simulink model "SystemDrivers"  (Simulink 8.3)
settings: Solver=ode45  StartTime=0.0  StopTime=50  RelTol=1e-4
model workspace (MAT data in the model file):
  MPS_ModuleName = 'ACC_Enhancement.ECR'
  variantInfo = VariabilitySupport
  variantInfo.name = 'ACCVarModel'
  variantInfo.featureModels = FeatureModel
  variantInfo.featureModels.id = '7NIE1o_FUkv'
  variantInfo.featureModels.name = 'ACCVars'
  variantInfo.featureModels.root = Feature
  variantInfo.featureModels.root.id = '7NIE1o_FUkw'
  variantInfo.featureModels.root.children(1) = Feature
  variantInfo.featureModels.root.children(1).id = '7NIE1o_FUxh'
  variantInfo.featureModels.root.children(1).name = 'SubjectProdFunction'
  variantInfo.featureModels.root.children(1).children(1) = Feature
  variantInfo.featureModels.root.children(1).children(1).id = '7NIE1o_FUzk'
  variantInfo.featureModels.root.children(1).children(1).name = 'S_ACC'
  variantInfo.featureModels.root.children(1).children(2) = Feature
  variantInfo.featureModels.root.children(1).children(2).id = '23v$6Q_kdyy'
  variantInfo.featureModels.root.children(1).children(2).name = 'S_ACC_SF'
  variantInfo.featureModels.root.children(1).children(3) = Feature
  variantInfo.featureModels.root.children(1).children(3).id = '7NIE1o_FUzr'
  variantInfo.featureModels.root.children(1).children(3).name = 'S_LearningACC'
  variantInfo.featureModels.root.children(1).children(4) = Feature
  variantInfo.featureModels.root.children(1).children(4).id = '23v$6Q_kdyD'
  variantInfo.featureModels.root.children(1).children(4).name = 'S_LearningACC_SF'
  variantInfo.featureModels.root.children(2) = Feature
  variantInfo.featureModels.root.children(2).id = '64YhESPcT$J'
  variantInfo.featureModels.root.children(2).name = 'SubjectDriverType'
  variantInfo.featureModels.root.children(2).children(1) = Feature
  variantInfo.featureModels.root.children(2).children(1).id = '64YhESPcT$S'
  variantInfo.featureModels.root.children(2).children(1).name = 'S_NormalDriver'
  variantInfo.featureModels.root.children(2).children(2) = Feature
  variantInfo.featureModels.root.children(2).children(2).id = '64YhESPcT$V'
  variantInfo.featureModels.root.children(2).children(2).name = 'S_ErraticDriver'
  variantInfo.featureModels.root.children(3) = Feature
  variantInfo.featureModels.root.children(3).id = '64YhESPd24W'
  variantInfo.featureModels.root.children(3).name = 'TargetProdFunction'
  variantInfo.featureModels.root.children(3).children(1) = Feature
  variantInfo.featureModels.root.children(3).children(1).id = '64YhESPd24Y'
  variantInfo.featureModels.root.children(3).children(1).name = 'T_ACC'
  variantInfo.featureModels.root.children(3).children(2) = Feature
  variantInfo.featureModels.root.children(3).children(2).id = '64YhESPd24Z'
  variantInfo.featureModels.root.children(3).children(2).name = 'T_LearningACC'
  variantInfo.featureModels.root.children(4) = Feature
  variantInfo.featureModels.root.children(4).id = '64YhESPd250'
  variantInfo.featureModels.root.children(4).name = 'TargetDriverType'
  variantInfo.featureModels.root.children(4).children(1) = Feature
  variantInfo.featureModels.root.children(4).children(1).id = '64YhESPd252'
  variantInfo.featureModels.root.children(4).children(1).name = 'T_NormalDriver'
  variantInfo.featureModels.root.children(4).children(2) = Feature
  variantInfo.featureModels.root.children(4).children(2).id = '64YhESPd253'
  variantInfo.featureModels.root.children(4).children(2).name = 'T_ErraticDriver'
  variantInfo.configModels(1) = VariantConfigurationModel
  variantInfo.configModels(1).id = '7NIE1o_G2gu'
  variantInfo.configModels(1).name = 'NormalACC'
  variantInfo.configModels(1).featureRef = MpsObjectRef
  variantInfo.configModels(1).featureRef.targetNodeId = '7NIE1o_FUkv'
  variantInfo.configModels(1).featureRef.resolveInfo = 'ACCVars'
  variantInfo.configModels(1).rootFeature = VariantSelectedFeature
  variantInfo.configModels(1).rootFeature.featureRef = MpsObjectRef
  variantInfo.configModels(1).rootFeature.featureRef.targetNodeId = '7NIE1o_FUkw'
  variantInfo.configModels(1).rootFeature.featureRef.resolveInfo = 'ACCVars_root'
  variantInfo.configModels(1).rootFeature.children(1) = VariantSelectedFeature
  variantInfo.configModels(1).rootFeature.children(1).featureRef = MpsObjectRef
  variantInfo.configModels(1).rootFeature.children(1).featureRef.targetNodeId = '7NIE1o_FUxh'
  variantInfo.configModels(1).rootFeature.children(1).featureRef.resolveInfo = 'SubjectProdFunction'
  variantInfo.configModels(1).rootFeature.children(1).children = VariantSelectedFeature
  variantInfo.configModels(1).rootFeature.children(1).children.featureRef = MpsObjectRef
  variantInfo.configModels(1).rootFeature.children(1).children.featureRef.targetNodeId = '7NIE1o_FUzk'
  variantInfo.configModels(1).rootFeature.children(1).children.featureRef.resolveInfo = 'S_ACC'
  variantInfo.configModels(1).rootFeature.children(2) = VariantSelectedFeature
  variantInfo.configModels(1).rootFeature.children(2).featureRef = MpsObjectRef
  variantInfo.configModels(1).rootFeature.children(2).featureRef.targetNodeId = '64YhESPcT$J'
  variantInfo.configModels(1).rootFeature.children(2).featureRef.resolveInfo = 'SubjectDriverType'
  variantInfo.configModels(1).rootFeature.children(2).children = VariantSelectedFeature
  variantInfo.configModels(1).rootFeature.children(2).children.featureRef = MpsObjectRef
  variantInfo.configModels(1).rootFeature.children(2).children.featureRef.targetNodeId = '64YhESPcT$S'
  variantInfo.configModels(1).rootFeature.children(2).children.featureRef.resolveInfo = 'S_NormalDriver'
  variantInfo.configModels(1).rootFeature.children(3) = VariantSelectedFeature
  variantInfo.configModels(1).rootFeature.children(3).featureRef = MpsObjectRef
  variantInfo.configModels(1).rootFeature.children(3).featureRef.targetNodeId = '64YhESPd24W'
  variantInfo.configModels(1).rootFeature.children(3).featureRef.resolveInfo = 'TargetProdFunction'
  variantInfo.configModels(1).rootFeature.children(3).children = VariantSelectedFeature
  variantInfo.configModels(1).rootFeature.children(3).children.featureRef = MpsObjectRef
  variantInfo.configModels(1).rootFeature.children(3).children.featureRef.targetNodeId = '64YhESPd24Y'
  variantInfo.configModels(1).rootFeature.children(3).children.featureRef.resolveInfo = 'T_ACC'
  variantInfo.configModels(1).rootFeature.children(4) = VariantSelectedFeature
  variantInfo.configModels(1).rootFeature.children(4).featureRef = MpsObjectRef
  variantInfo.configModels(1).rootFeature.children(4).featureRef.targetNodeId = '64YhESPd250'
  variantInfo.configModels(1).rootFeature.children(4).featureRef.resolveInfo = 'TargetDriverType'
  variantInfo.configModels(1).rootFeature.children(4).children = VariantSelectedFeature
  variantInfo.configModels(1).rootFeature.children(4).children.featureRef = MpsObjectRef
  variantInfo.configModels(1).rootFeature.children(4).children.featureRef.targetNodeId = '64YhESPd252'
  variantInfo.configModels(1).rootFeature.children(4).children.featureRef.resolveInfo = 'T_NormalDriver'
  variantInfo.configModels(2) = VariantConfigurationModel
  variantInfo.configModels(2).id = '23v$6Q_kdSe'
  variantInfo.configModels(2).name = 'NormalACC_SF'
  variantInfo.configModels(2).featureRef = MpsObjectRef
  variantInfo.configModels(2).featureRef.targetNodeId = '7NIE1o_FUkv'
  variantInfo.configModels(2).featureRef.resolveInfo = 'ACCVars'
  variantInfo.configModels(2).rootFeature = VariantSelectedFeature
  variantInfo.configModels(2).rootFeature.featureRef = MpsObjectRef
  variantInfo.configModels(2).rootFeature.featureRef.targetNodeId = '7NIE1o_FUkw'
  variantInfo.configModels(2).rootFeature.featureRef.resolveInfo = 'ACCVars_root'
  variantInfo.configModels(2).rootFeature.children(1) = VariantSelectedFeature
  variantInfo.configModels(2).rootFeature.children(1).featureRef = MpsObjectRef
  variantInfo.configModels(2).rootFeature.children(1).featureRef.targetNodeId = '7NIE1o_FUxh'
  variantInfo.configModels(2).rootFeature.children(1).featureRef.resolveInfo = 'SubjectProdFunction'
  variantInfo.configModels(2).rootFeature.children(1).children = VariantSelectedFeature
  variantInfo.configModels(2).rootFeature.children(1).children.featureRef = MpsObjectRef
  variantInfo.configModels(2).rootFeature.children(1).children.featureRef.targetNodeId = '23v$6Q_kdyy'
  variantInfo.configModels(2).rootFeature.children(1).children.featureRef.resolveInfo = 'S_ACC_SF'
  variantInfo.configModels(2).rootFeature.children(2) = VariantSelectedFeature
  variantInfo.configModels(2).rootFeature.children(2).featureRef = MpsObjectRef
  variantInfo.configModels(2).rootFeature.children(2).featureRef.targetNodeId = '64YhESPcT$J'
  variantInfo.configModels(2).rootFeature.children(2).featureRef.resolveInfo = 'SubjectDriverType'
  variantInfo.configModels(2).rootFeature.children(2).children = VariantSelectedFeature
  variantInfo.configModels(2).rootFeature.children(2).children.featureRef = MpsObjectRef
  variantInfo.configModels(2).rootFeature.children(2).children.featureRef.targetNodeId = '64YhESPcT$S'
  variantInfo.configModels(2).rootFeature.children(2).children.featureRef.resolveInfo = 'S_NormalDriver'
  variantInfo.configModels(2).rootFeature.children(3) = VariantSelectedFeature
  variantInfo.configModels(2).rootFeature.children(3).featureRef = MpsObjectRef
  variantInfo.configModels(2).rootFeature.children(3).featureRef.targetNodeId = '64YhESPd24W'
  variantInfo.configModels(2).rootFeature.children(3).featureRef.resolveInfo = 'TargetProdFunction'
  variantInfo.configModels(2).rootFeature.children(3).children = VariantSelectedFeature
  variantInfo.configModels(2).rootFeature.children(3).children.featureRef = MpsObjectRef
  variantInfo.configModels(2).rootFeature.children(3).children.featureRef.targetNodeId = '64YhESPd24Y'
  variantInfo.configModels(2).rootFeature.children(3).children.featureRef.resolveInfo = 'T_ACC'
  variantInfo.configModels(2).rootFeature.children(4) = VariantSelectedFeature
  variantInfo.configModels(2).rootFeature.children(4).featureRef = MpsObjectRef
  variantInfo.configModels(2).rootFeature.children(4).featureRef.targetNodeId = '64YhESPd250'
  variantInfo.configModels(2).rootFeature.children(4).featureRef.resolveInfo = 'TargetDriverType'
  variantInfo.configModels(2).rootFeature.children(4).children = VariantSelectedFeature
  variantInfo.configModels(2).rootFeature.children(4).children.featureRef = MpsObjectRef
  variantInfo.configModels(2).rootFeature.children(4).children.featureRef.targetNodeId = '64YhESPd252'
  variantInfo.configModels(2).rootFeature.children(4).children.featureRef.resolveInfo = 'T_NormalDriver'
  variantInfo.configModels(3) = VariantConfigurationModel
  variantInfo.configModels(3).id = '7NIE1o_FUDp'
  variantInfo.configModels(3).name = 'ErraticDriverACC'
  variantInfo.configModels(3).featureRef = MpsObjectRef
  variantInfo.configModels(3).featureRef.targetNodeId = '7NIE1o_FUkv'
  variantInfo.configModels(3).featureRef.resolveInfo = 'ACCVars'
  variantInfo.configModels(3).rootFeature = VariantSelectedFeature
  variantInfo.configModels(3).rootFeature.featureRef = MpsObjectRef
  variantInfo.configModels(3).rootFeature.featureRef.targetNodeId = '7NIE1o_FUkw'
  variantInfo.configModels(3).rootFeature.featureRef.resolveInfo = 'ACCVars_root'
  variantInfo.configModels(3).rootFeature.children(1) = VariantSelectedFeature
  variantInfo.configModels(3).rootFeature.children(1).featureRef = MpsObjectRef
  variantInfo.configModels(3).rootFeature.children(1).featureRef.targetNodeId = '7NIE1o_FUxh'
  variantInfo.configModels(3).rootFeature.children(1).featureRef.resolveInfo = 'SubjectProdFunction'
  variantInfo.configModels(3).rootFeature.children(1).children = VariantSelectedFeature
  variantInfo.configModels(3).rootFeature.children(1).children.featureRef = MpsObjectRef
  variantInfo.configModels(3).rootFeature.children(1).children.featureRef.targetNodeId = '7NIE1o_FUzk'
  variantInfo.configModels(3).rootFeature.children(1).children.featureRef.resolveInfo = 'S_ACC'
  variantInfo.configModels(3).rootFeature.children(2) = VariantSelectedFeature
  variantInfo.configModels(3).rootFeature.children(2).featureRef = MpsObjectRef
  variantInfo.configModels(3).rootFeature.children(2).featureRef.targetNodeId = '64YhESPcT$J'
  variantInfo.configModels(3).rootFeature.children(2).featureRef.resolveInfo = 'SubjectDriverType'
  variantInfo.configModels(3).rootFeature.children(2).children = VariantSelectedFeature
  variantInfo.configModels(3).rootFeature.children(2).children.featureRef = MpsObjectRef
  variantInfo.configModels(3).rootFeature.children(2).children.featureRef.targetNodeId = '64YhESPcT$S'
  variantInfo.configModels(3).rootFeature.children(2).children.featureRef.resolveInfo = 'S_NormalDriver'
  variantInfo.configModels(3).rootFeature.children(3) = VariantSelectedFeature
  variantInfo.configModels(3).rootFeature.children(3).featureRef = MpsObjectRef
  variantInfo.configModels(3).rootFeature.children(3).featureRef.targetNodeId = '64YhESPd24W'
  variantInfo.configModels(3).rootFeature.children(3).featureRef.resolveInfo = 'TargetProdFunction'
  variantInfo.configModels(3).rootFeature.children(3).children = VariantSelectedFeature
  variantInfo.configModels(3).rootFeature.children(3).children.featureRef = MpsObjectRef
  variantInfo.configModels(3).rootFeature.children(3).children.featureRef.targetNodeId = '64YhESPd24Y'
  variantInfo.configModels(3).rootFeature.children(3).children.featureRef.resolveInfo = 'T_ACC'
  variantInfo.configModels(3).rootFeature.children(4) = VariantSelectedFeature
  variantInfo.configModels(3).rootFeature.children(4).featureRef = MpsObjectRef
  variantInfo.configModels(3).rootFeature.children(4).featureRef.targetNodeId = '64YhESPd250'
  variantInfo.configModels(3).rootFeature.children(4).featureRef.resolveInfo = 'TargetDriverType'
  variantInfo.configModels(3).rootFeature.children(4).children = VariantSelectedFeature
  variantInfo.configModels(3).rootFeature.children(4).children.featureRef = MpsObjectRef
  variantInfo.configModels(3).rootFeature.children(4).children.featureRef.targetNodeId = '64YhESPd253'
  variantInfo.configModels(3).rootFeature.children(4).children.featureRef.resolveInfo = 'T_ErraticDriver'
  variantInfo.configModels(4) = VariantConfigurationModel
  variantInfo.configModels(4).id = '23v$6Q_kef3'
  variantInfo.configModels(4).name = 'ErraticDriverACC_SF'
  variantInfo.configModels(4).featureRef = MpsObjectRef
  variantInfo.configModels(4).featureRef.targetNodeId = '7NIE1o_FUkv'
  variantInfo.configModels(4).featureRef.resolveInfo = 'ACCVars'
  variantInfo.configModels(4).rootFeature = VariantSelectedFeature
  variantInfo.configModels(4).rootFeature.featureRef = MpsObjectRef
  variantInfo.configModels(4).rootFeature.featureRef.targetNodeId = '7NIE1o_FUkw'
  variantInfo.configModels(4).rootFeature.featureRef.resolveInfo = 'ACCVars_root'
  variantInfo.configModels(4).rootFeature.children(1) = VariantSelectedFeature
  variantInfo.configModels(4).rootFeature.children(1).featureRef = MpsObjectRef
  variantInfo.configModels(4).rootFeature.children(1).featureRef.targetNodeId = '7NIE1o_FUxh'
  variantInfo.configModels(4).rootFeature.children(1).featureRef.resolveInfo = 'SubjectProdFunction'
  variantInfo.configModels(4).rootFeature.children(1).children = VariantSelectedFeature
  variantInfo.configModels(4).rootFeature.children(1).children.featureRef = MpsObjectRef
  variantInfo.configModels(4).rootFeature.children(1).children.featureRef.targetNodeId = '23v$6Q_kdyy'
  variantInfo.configModels(4).rootFeature.children(1).children.featureRef.resolveInfo = 'S_ACC_SF'
  variantInfo.configModels(4).rootFeature.children(2) = VariantSelectedFeature
  variantInfo.configModels(4).rootFeature.children(2).featureRef = MpsObjectRef
  variantInfo.configModels(4).rootFeature.children(2).featureRef.targetNodeId = '64YhESPcT$J'
  variantInfo.configModels(4).rootFeature.children(2).featureRef.resolveInfo = 'SubjectDriverType'
  variantInfo.configModels(4).rootFeature.children(2).children = VariantSelectedFeature
  variantInfo.configModels(4).rootFeature.children(2).children.featureRef = MpsObjectRef
  variantInfo.configModels(4).rootFeature.children(2).children.featureRef.targetNodeId = '64YhESPcT$S'
  variantInfo.configModels(4).rootFeature.children(2).children.featureRef.resolveInfo = 'S_NormalDriver'
  variantInfo.configModels(4).rootFeature.children(3) = VariantSelectedFeature
  variantInfo.configModels(4).rootFeature.children(3).featureRef = MpsObjectRef
  variantInfo.configModels(4).rootFeature.children(3).featureRef.targetNodeId = '64YhESPd24W'
  variantInfo.configModels(4).rootFeature.children(3).featureRef.resolveInfo = 'TargetProdFunction'
  variantInfo.configModels(4).rootFeature.children(3).children = VariantSelectedFeature
  variantInfo.configModels(4).rootFeature.children(3).children.featureRef = MpsObjectRef
  variantInfo.configModels(4).rootFeature.children(3).children.featureRef.targetNodeId = '64YhESPd24Y'
  variantInfo.configModels(4).rootFeature.children(3).children.featureRef.resolveInfo = 'T_ACC'
  variantInfo.configModels(4).rootFeature.children(4) = VariantSelectedFeature
  variantInfo.configModels(4).rootFeature.children(4).featureRef = MpsObjectRef
  variantInfo.configModels(4).rootFeature.children(4).featureRef.targetNodeId = '64YhESPd250'
  variantInfo.configModels(4).rootFeature.children(4).featureRef.resolveInfo = 'TargetDriverType'
  variantInfo.configModels(4).rootFeature.children(4).children = VariantSelectedFeature
  variantInfo.configModels(4).rootFeature.children(4).children.featureRef = MpsObjectRef
  variantInfo.configModels(4).rootFeature.children(4).children.featureRef.targetNodeId = '64YhESPd253'
  variantInfo.configModels(4).rootFeature.children(4).children.featureRef.resolveInfo = 'T_ErraticDriver'
  variantInfo.configModels(5) = VariantConfigurationModel
  variantInfo.configModels(5).id = '7NIE1o_FUF3'
  variantInfo.configModels(5).name = 'ErraticDriverACCFix'
  variantInfo.configModels(5).featureRef = MpsObjectRef
  variantInfo.configModels(5).featureRef.targetNodeId = '7NIE1o_FUkv'
  variantInfo.configModels(5).featureRef.resolveInfo = 'ACCVars'
  variantInfo.configModels(5).rootFeature = VariantSelectedFeature
  variantInfo.configModels(5).rootFeature.featureRef = MpsObjectRef
  variantInfo.configModels(5).rootFeature.featureRef.targetNodeId = '7NIE1o_FUkw'
  variantInfo.configModels(5).rootFeature.featureRef.resolveInfo = 'ACCVars_root'
  variantInfo.configModels(5).rootFeature.children(1) = VariantSelectedFeature
  variantInfo.configModels(5).rootFeature.children(1).featureRef = MpsObjectRef
  variantInfo.configModels(5).rootFeature.children(1).featureRef.targetNodeId = '7NIE1o_FUxh'
  variantInfo.configModels(5).rootFeature.children(1).featureRef.resolveInfo = 'SubjectProdFunction'
  variantInfo.configModels(5).rootFeature.children(1).children = VariantSelectedFeature
  variantInfo.configModels(5).rootFeature.children(1).children.featureRef = MpsObjectRef
  variantInfo.configModels(5).rootFeature.children(1).children.featureRef.targetNodeId = '7NIE1o_FUzr'
  variantInfo.configModels(5).rootFeature.children(1).children.featureRef.resolveInfo = 'S_LearningACC'
  variantInfo.configModels(5).rootFeature.children(2) = VariantSelectedFeature
  variantInfo.configModels(5).rootFeature.children(2).featureRef = MpsObjectRef
  variantInfo.configModels(5).rootFeature.children(2).featureRef.targetNodeId = '64YhESPcT$J'
  variantInfo.configModels(5).rootFeature.children(2).featureRef.resolveInfo = 'SubjectDriverType'
  variantInfo.configModels(5).rootFeature.children(2).children = VariantSelectedFeature
  variantInfo.configModels(5).rootFeature.children(2).children.featureRef = MpsObjectRef
  variantInfo.configModels(5).rootFeature.children(2).children.featureRef.targetNodeId = '64YhESPcT$S'
  variantInfo.configModels(5).rootFeature.children(2).children.featureRef.resolveInfo = 'S_NormalDriver'
  variantInfo.configModels(5).rootFeature.children(3) = VariantSelectedFeature
  variantInfo.configModels(5).rootFeature.children(3).featureRef = MpsObjectRef
  variantInfo.configModels(5).rootFeature.children(3).featureRef.targetNodeId = '64YhESPd24W'
  variantInfo.configModels(5).rootFeature.children(3).featureRef.resolveInfo = 'TargetProdFunction'
  variantInfo.configModels(5).rootFeature.children(3).children = VariantSelectedFeature
  variantInfo.configModels(5).rootFeature.children(3).children.featureRef = MpsObjectRef
  variantInfo.configModels(5).rootFeature.children(3).children.featureRef.targetNodeId = '64YhESPd24Y'
  variantInfo.configModels(5).rootFeature.children(3).children.featureRef.resolveInfo = 'T_ACC'
  variantInfo.configModels(5).rootFeature.children(4) = VariantSelectedFeature
  variantInfo.configModels(5).rootFeature.children(4).featureRef = MpsObjectRef
  variantInfo.configModels(5).rootFeature.children(4).featureRef.targetNodeId = '64YhESPd250'
  variantInfo.configModels(5).rootFeature.children(4).featureRef.resolveInfo = 'TargetDriverType'
  variantInfo.configModels(5).rootFeature.children(4).children = VariantSelectedFeature
  variantInfo.configModels(5).rootFeature.children(4).children.featureRef = MpsObjectRef
  variantInfo.configModels(5).rootFeature.children(4).children.featureRef.targetNodeId = '64YhESPd253'
  variantInfo.configModels(5).rootFeature.children(4).children.featureRef.resolveInfo = 'T_ErraticDriver'
  variantInfo.configModels(6) = VariantConfigurationModel
  variantInfo.configModels(6).id = '23v$6Q_kdWi'
  variantInfo.configModels(6).name = 'ErraticDriverACCFix_SF'
  variantInfo.configModels(6).featureRef = MpsObjectRef
  variantInfo.configModels(6).featureRef.targetNodeId = '7NIE1o_FUkv'
  variantInfo.configModels(6).featureRef.resolveInfo = 'ACCVars'
  variantInfo.configModels(6).rootFeature = VariantSelectedFeature
  variantInfo.configModels(6).rootFeature.featureRef = MpsObjectRef
  variantInfo.configModels(6).rootFeature.featureRef.targetNodeId = '7NIE1o_FUkw'
  variantInfo.configModels(6).rootFeature.featureRef.resolveInfo = 'ACCVars_root'
  variantInfo.configModels(6).rootFeature.children(1) = VariantSelectedFeature
  variantInfo.configModels(6).rootFeature.children(1).featureRef = MpsObjectRef
  variantInfo.configModels(6).rootFeature.children(1).featureRef.targetNodeId = '7NIE1o_FUxh'
  variantInfo.configModels(6).rootFeature.children(1).featureRef.resolveInfo = 'SubjectProdFunction'
  variantInfo.configModels(6).rootFeature.children(1).children = VariantSelectedFeature
  variantInfo.configModels(6).rootFeature.children(1).children.featureRef = MpsObjectRef
  variantInfo.configModels(6).rootFeature.children(1).children.featureRef.targetNodeId = '23v$6Q_kdyD'
  variantInfo.configModels(6).rootFeature.children(1).children.featureRef.resolveInfo = 'S_LearningACC_SF'
  variantInfo.configModels(6).rootFeature.children(2) = VariantSelectedFeature
  variantInfo.configModels(6).rootFeature.children(2).featureRef = MpsObjectRef
  variantInfo.configModels(6).rootFeature.children(2).featureRef.targetNodeId = '64YhESPcT$J'
  variantInfo.configModels(6).rootFeature.children(2).featureRef.resolveInfo = 'SubjectDriverType'
  variantInfo.configModels(6).rootFeature.children(2).children = VariantSelectedFeature
  variantInfo.configModels(6).rootFeature.children(2).children.featureRef = MpsObjectRef
  variantInfo.configModels(6).rootFeature.children(2).children.featureRef.targetNodeId = '64YhESPcT$S'
  variantInfo.configModels(6).rootFeature.children(2).children.featureRef.resolveInfo = 'S_NormalDriver'
  variantInfo.configModels(6).rootFeature.children(3) = VariantSelectedFeature
  variantInfo.configModels(6).rootFeature.children(3).featureRef = MpsObjectRef
  variantInfo.configModels(6).rootFeature.children(3).featureRef.targetNodeId = '64YhESPd24W'
  variantInfo.configModels(6).rootFeature.children(3).featureRef.resolveInfo = 'TargetProdFunction'
  variantInfo.configModels(6).rootFeature.children(3).children = VariantSelectedFeature
  variantInfo.configModels(6).rootFeature.children(3).children.featureRef = MpsObjectRef
  variantInfo.configModels(6).rootFeature.children(3).children.featureRef.targetNodeId = '64YhESPd24Y'
  variantInfo.configModels(6).rootFeature.children(3).children.featureRef.resolveInfo = 'T_ACC'
  variantInfo.configModels(6).rootFeature.children(4) = VariantSelectedFeature
  variantInfo.configModels(6).rootFeature.children(4).featureRef = MpsObjectRef
  variantInfo.configModels(6).rootFeature.children(4).featureRef.targetNodeId = '64YhESPd250'
  variantInfo.configModels(6).rootFeature.children(4).featureRef.resolveInfo = 'TargetDriverType'
  variantInfo.configModels(6).rootFeature.children(4).children = VariantSelectedFeature
  variantInfo.configModels(6).rootFeature.children(4).children.featureRef = MpsObjectRef
  variantInfo.configModels(6).rootFeature.children(4).children.featureRef.targetNodeId = '64YhESPd253'
  variantInfo.configModels(6).rootFeature.children(4).children.featureRef.resolveInfo = 'T_ErraticDriver'
undefined symbols (not defined in the file): Engine, Trans
libraries: simulink x2
settings Model: Creator=swami  LastModifiedBy=swami
settings SolverCC: ShapePreserveControl=EnableAll  ZeroCrossControl=EnableAll
settings DataIOCC: SignalLoggingSaveFormat=Dataset
settings DebuggingCC: UnderspecifiedInitializationDetection=Simplified  MergeDetectMultiDrivingBlocksExec=error  FrameProcessingCompatibilityMsg=error  StateNameClashWarn=none
settings ModelReferenceCC: UpdateModelReferenceTargets=Force
settings GRTTargetCC: CombineOutputUpdateFcns=on  GRTInterface=off
settings ConfigComp: CovMetricSettings=dw  CovHtmlReporting=on  CovSaveCumulativeToWorkspaceVar=on  CovSaveSingleToWorkspaceVar=on  CovModelRefEnable=Off  CovExternalEMLEnable=off  CovSFcnEnable=off

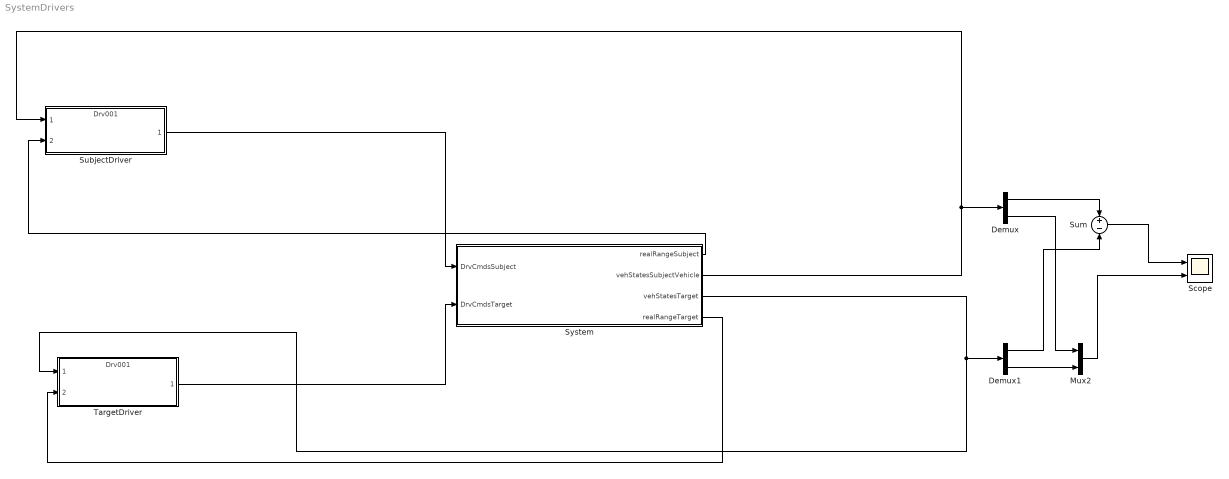
== system SystemDrivers ==
  Demux : Demux  Outputs=2
  Demux1 : Demux  Outputs=2
  Mux2 : Mux  Inputs=2
  Scope : Scope  NumInputPorts=2
  SubjectDriver : ModelReference  ModelNameDialog=Drv001  ParameterArgumentNames=pDrv  ParameterArgumentValues=DrvSubject  SimulationMode=Normal  Variant=on  OverrideUsingVariant=ECR1_varDrv001  ModelReferenceVersion=1.22  CopyOfModelName=Drv001  DefaultDataLogging=on
      settings: AttributesFormatString=%<ActiveVariant>
  Sum : Sum  Inputs=+-
  System : Subsystem
  TargetDriver : ModelReference  ModelNameDialog=Drv001  ParameterArgumentNames=pDrv  ParameterArgumentValues=DrvTarget  SimulationMode=Normal  Variant=on  OverrideUsingVariant=ECR1_varDrv001  ModelReferenceVersion=1.22  CopyOfModelName=Drv001  DefaultDataLogging=on
      settings: AttributesFormatString=%<ActiveVariant>
  wires:
  Demux/1 -> Sum/1
  Demux1/1 -> Sum/2
  Demux/2 -> Mux2/1
  Demux1/2 -> Mux2/2
  Mux2/1 -> Scope/2
  Sum/1 -> Scope/1
  System/2(vehStatesSubjectVehicle) -> SubjectDriver/1, Demux/1
  SubjectDriver/1 -> System/1(DrvCmdsSubject)
  TargetDriver/1 -> System/2(DrvCmdsTarget)
  System/1(realRangeSubject) -> SubjectDriver/2
  System/4(realRangeTarget) -> TargetDriver/2
  System/3(vehStatesTarget) -> TargetDriver/1, Demux1/1

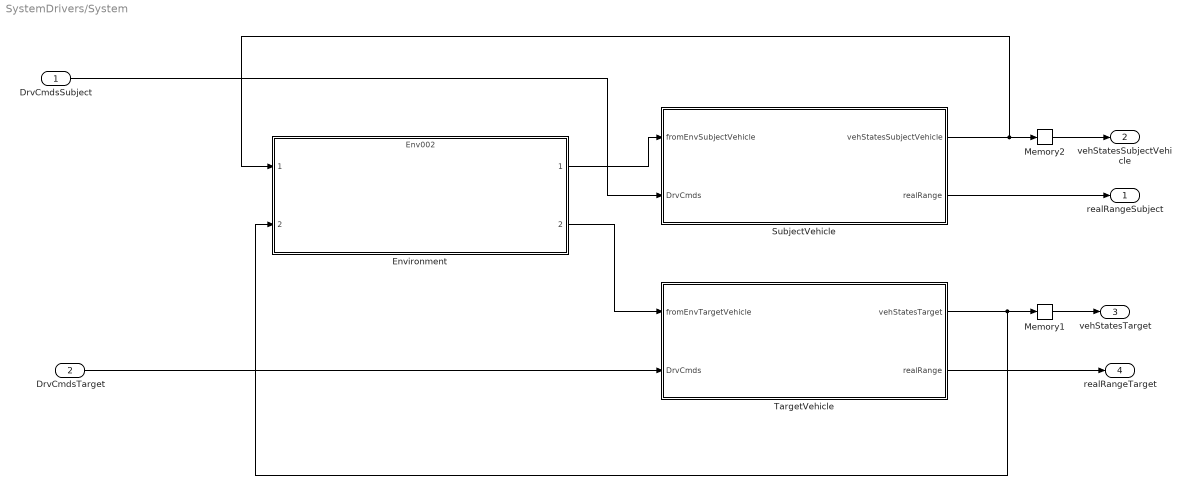
== system SystemDrivers/System ==
  DrvCmdsSubject : Inport  OutDataTypeStr=double
  DrvCmdsTarget : Inport  Port=2
  Environment : ModelReference  ModelNameDialog=Env002  SimulationMode=Normal  Variant=on  OverrideUsingVariant=ECR1_varEnv002  ModelReferenceVersion=1.10  CopyOfModelName=Env002  DefaultDataLogging=on
      settings: AttributesFormatString=%<ActiveVariant>
  Memory1 : Memory
  Memory2 : Memory
  SubjectVehicle : Subsystem
  TargetVehicle : Subsystem
  realRangeSubject : Outport
  vehStatesSubjectVehicle : Outport  Port=2
  vehStatesTarget : Outport  Port=3
  realRangeTarget : Outport  Port=4
  wires:
  TargetVehicle/1(vehStatesTarget) -> Environment/2, Memory1/1
  Environment/2 -> TargetVehicle/1(fromEnvTargetVehicle)
  Environment/1 -> SubjectVehicle/1(fromEnvSubjectVehicle)
  SubjectVehicle/1(vehStatesSubjectVehicle) -> Environment/1, Memory2/1
  SubjectVehicle/2(realRange) -> realRangeSubject/1
  TargetVehicle/2(realRange) -> realRangeTarget/1
  DrvCmdsTarget/1 -> TargetVehicle/2(DrvCmds)
  DrvCmdsSubject/1 -> SubjectVehicle/2(DrvCmds)
  Memory2/1 -> vehStatesSubjectVehicle/1
  Memory1/1 -> vehStatesTarget/1

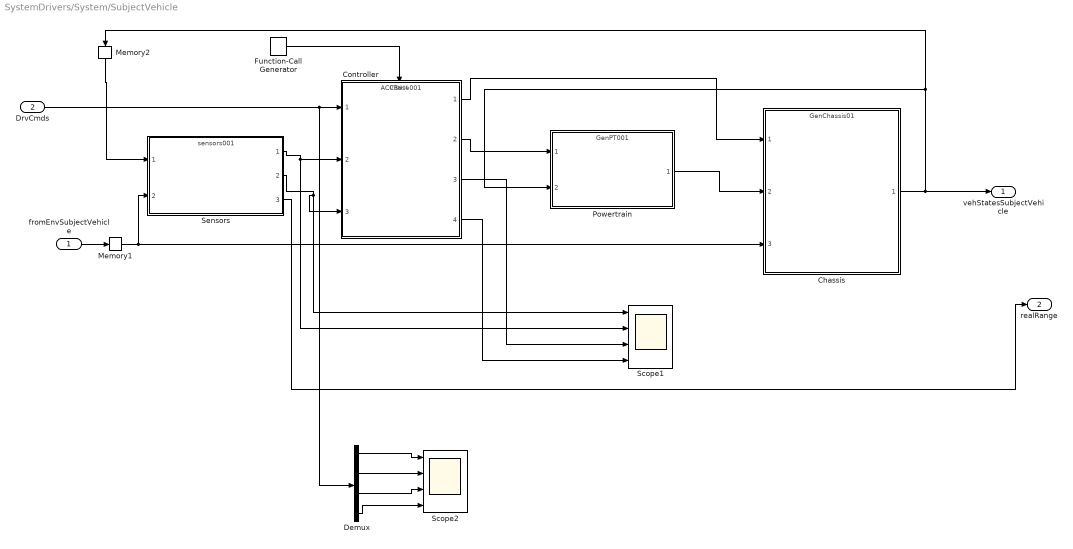
== system SystemDrivers/System/SubjectVehicle ==
  fromEnvSubjectVehicle : Inport
  DrvCmds : Inport  Port=2
  Chassis : ModelReference  ModelNameDialog=GenChassis01  ParameterArgumentNames=Chassis  ParameterArgumentValues=ChassisSubject  SimulationMode=Normal  Variant=on  OverrideUsingVariant=ECR1_varChassis01  ModelReferenceVersion=1.19  CopyOfModelName=GenChassis01  DefaultDataLogging=on
      settings: AttributesFormatString=%<ActiveVariant>
  Controller : ModelReference  ModelNameDialog=ACCBase001  ParameterArgumentNames=pACC  ParameterArgumentValues=pACCBase  SimulationMode=Normal  Variant=on  OverrideUsingVariant=ECR1_varACCBase001  ModelReferenceVersion=1.94  CopyOfModelName=ACCBase001  DefaultDataLogging=on  TriggerPortName=Trigger  TriggerPortTriggerType=function-call  TriggerPortStatesWhenEnabling=held
      settings: AttributesFormatString=%<ActiveVariant>
  Demux : Demux
  Function-Call Generator : simulink/Ports & Subsystems/Function-Call Generator  sample_time=0.1  numberOfIterations=1
  Memory1 : Memory
  Memory2 : Memory
  Powertrain : ModelReference  ModelNameDialog=GenPT001  ParameterArgumentNames=Trans,Engine  ParameterArgumentValues=Trans,Engine  SimulationMode=Normal  Variant=on  OverrideUsingVariant=ECR1_varGenPT001  ModelReferenceVersion=1.23  CopyOfModelName=GenPT001  DefaultDataLogging=on
      settings: AttributesFormatString=%<ActiveVariant>
  Scope1 : Scope  NumInputPorts=4
  Scope2 : Scope  NumInputPorts=4
  Sensors : ModelReference  ModelNameDialog=sensors001  SimulationMode=Normal  Variant=on  OverrideUsingVariant=ECR1_varSensor001  ModelReferenceVersion=1.21  CopyOfModelName=sensors001  DefaultDataLogging=on
      settings: AttributesFormatString=%<ActiveVariant>
  vehStatesSubjectVehicle : Outport
  realRange : Outport  Port=2
  wires:
  Chassis/1 -> Powertrain/2, Memory2/1, vehStatesSubjectVehicle/1
  Controller/2 -> Powertrain/1
  Powertrain/1 -> Chassis/2
  Controller/1 -> Chassis/1
  Sensors/1 -> Scope1/2, Controller/2
  Sensors/2 -> Controller/3, Scope1/1
  DrvCmds/1 -> Demux/1, Controller/1
  Memory2/1 -> Sensors/1
  fromEnvSubjectVehicle/1 -> Memory1/1
  Memory1/1 -> Sensors/2, Chassis/3
  Function-Call Generator/1 -> Controller/Trigger
  Controller/3 -> Scope1/3
  Controller/4 -> Scope1/4
  Sensors/3 -> realRange/1
  Demux/2 -> Scope2/2
  Demux/3 -> Scope2/3
  Demux/1 -> Scope2/1
  Demux/4 -> Scope2/4

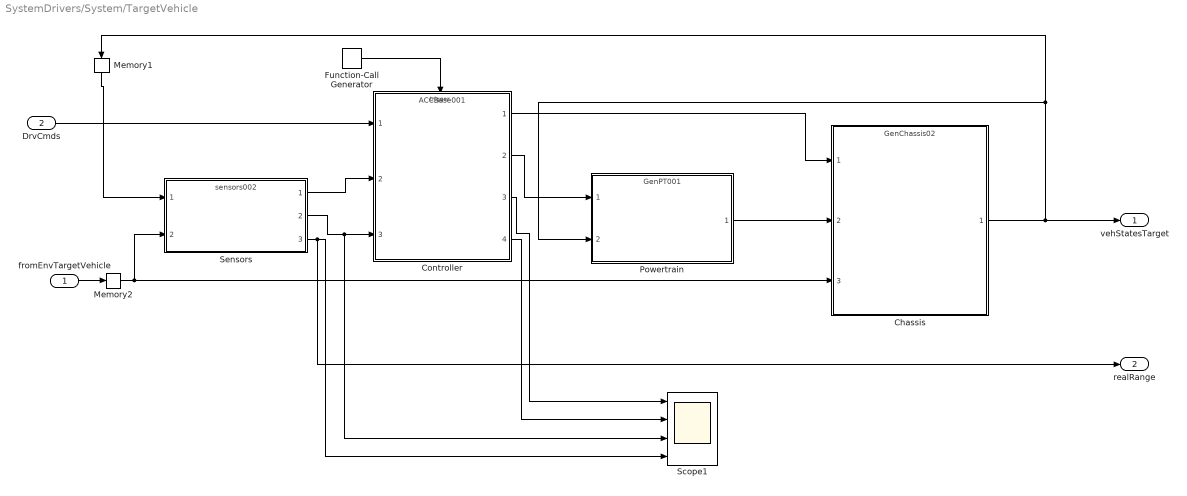
== system SystemDrivers/System/TargetVehicle ==
  fromEnvTargetVehicle : Inport
  DrvCmds : Inport  Port=2
  Chassis : ModelReference  ModelNameDialog=GenChassis02  ParameterArgumentNames=Chassis  ParameterArgumentValues=ChassisTarget  SimulationMode=Normal  Variant=on  OverrideUsingVariant=ECR1_varChassis02  ModelReferenceVersion=1.19  CopyOfModelName=GenChassis02  DefaultDataLogging=on
      settings: AttributesFormatString=%<ActiveVariant>
  Controller : ModelReference  ModelNameDialog=ACCBase001  ParameterArgumentNames=pACC  ParameterArgumentValues=pACCBase  SimulationMode=Normal  Variant=on  OverrideUsingVariant=ECR1_var0005  ModelReferenceVersion=1.94  CopyOfModelName=ACCBase001  DefaultDataLogging=on  TriggerPortName=Trigger  TriggerPortTriggerType=function-call  TriggerPortStatesWhenEnabling=held
      settings: AttributesFormatString=%<ActiveVariant>
  Function-Call Generator : simulink/Ports & Subsystems/Function-Call Generator  sample_time=0.1  numberOfIterations=1
  Memory1 : Memory
  Memory2 : Memory
  Powertrain : ModelReference  ModelNameDialog=GenPT001  ParameterArgumentNames=Trans,Engine  ParameterArgumentValues=Trans,Engine  SimulationMode=Normal  Variant=on  OverrideUsingVariant=ECR1_varGenPT001  ModelReferenceVersion=1.23  CopyOfModelName=GenPT001  DefaultDataLogging=on
      settings: AttributesFormatString=%<ActiveVariant>
  Scope1 : Scope  NumInputPorts=4
  Sensors : ModelReference  ModelNameDialog=sensors002  SimulationMode=Normal  Variant=on  OverrideUsingVariant=varObject1  ModelReferenceVersion=1.19  CopyOfModelName=sensors002  DefaultDataLogging=on
      settings: AttributesFormatString=%<ActiveVariant>
  vehStatesTarget : Outport
  realRange : Outport  Port=2
  wires:
  Sensors/2 -> Scope1/3, Controller/3
  Sensors/1 -> Controller/2
  DrvCmds/1 -> Controller/1
  Controller/1 -> Chassis/1
  Powertrain/1 -> Chassis/2
  Controller/2 -> Powertrain/1
  fromEnvTargetVehicle/1 -> Memory2/1
  Chassis/1 -> vehStatesTarget/1, Memory1/1, Powertrain/2
  Memory1/1 -> Sensors/1
  Memory2/1 -> Sensors/2, Chassis/3
  Function-Call Generator/1 -> Controller/Trigger
  Controller/3 -> Scope1/1
  Controller/4 -> Scope1/2
  Sensors/3 -> realRange/1, Scope1/4
